simulink model "SalirClaseConObstaculos"  (R2022b)
settings: Solver=FixedStepAuto  StartTime=0.0  StopTime=inf  RelTol=1e-3  EnableMultiTasking=on
model workspace (MAT data in the model file):
  d = Simulink.Parameter
  d.Value = 0.22
  d.DataType = 'double'
  d.Complexity = 'real'
  d.Dimensions = [1 1]
libraries: robotalgslib x1
settings Model: ExtModeTrigDuration=2  Creator=Usuario_UMA  LastModifiedBy=dar.io
settings OptimizationCC: EnhancedBackFolding=on  PassReuseOutputArgsAs=Individual arguments  ZeroExternalMemoryAtStartup=off  ZeroInternalMemoryAtStartup=off  MaxStackSize=64  OptimizeBlockOrder=speed  DifferentSizesBufferReuse=on  OptimizationCustomize=off  EfficientTunableParamExpr=on
settings DebuggingCC: ParameterTunabilityLossMsg=error
settings HardwareCC: ProdBitPerInt=16  ProdBitPerPointer=16  ProdBitPerSizeT=16  ProdBitPerPtrDiffT=16  ProdLargestAtomicFloat=None  ProdWordSize=8  ProdHWDeviceType=Atmel->AVR  UseEmbeddedCoderFeatures=off  UseSimulinkCoderFeatures=off
settings SFSimCC: MATLABDynamicMemAlloc=off
settings RTWCC: Description=Embedded Coder  SystemTargetFile=ert.tlc  HardwareBoard=Arduino Mega 2560  TLCOptions=-aInlineSetEventsForThisBaseRateFcn=TLC_FALSE -aSuppressMultiTaskScheduler=TLC_FALSE -aRateBasedStepFcn=1  TemplateMakefile=ert_default_tmf  Toolchain=Arduino AVR  BuildConfiguration=Faster Runs
settings CodeAppCC: ForceParamTrailComments=on  IgnoreCustomStorageClasses=off  OperatorAnnotations=on  SimulinkDataObjDesc=on  SFDataObjDesc=on  MangleLength=10  InsertBlockDesc=on
settings ERTTargetCC: SupportContinuousTime=on  SupportNonInlinedSFcns=on  SupportVariableSizeSignals=on  ExtModeTransport=3  ExtModeStaticAlloc=on  ExtModeAutomaticAllocSize=off  ExtModeStaticAllocSize=2048  ExtModeMexFile=ext_xcp  ExtModeIntrfLevel=Level2 - Open

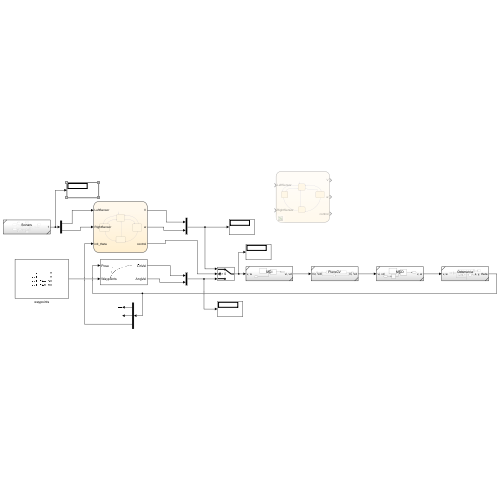
[thumbnail: Simulink's stored preview of the top-level diagram]
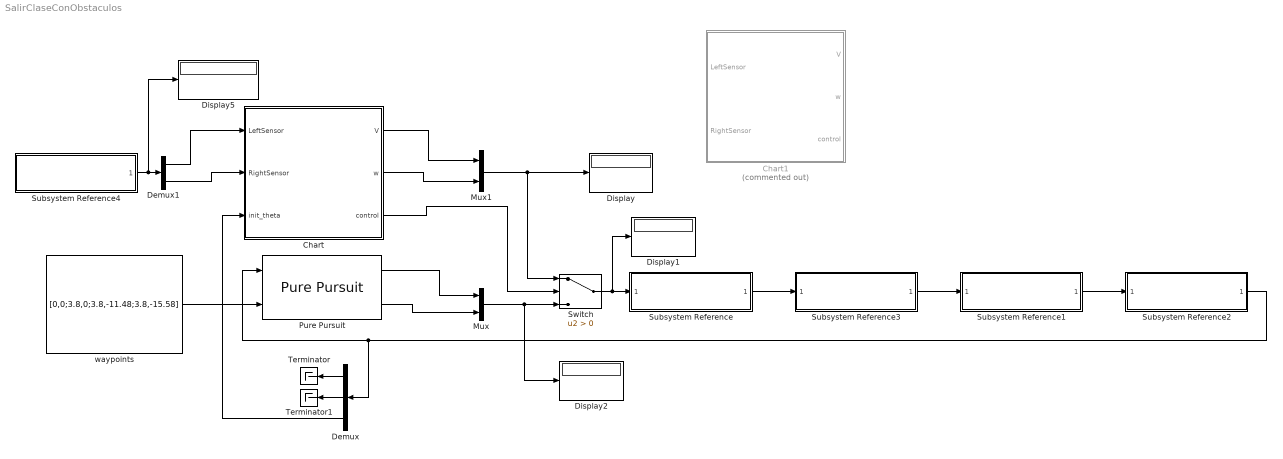
== system SalirClaseConObstaculos ==
  Chart : Stateflow chart  TreatAsAtomicUnit=on
  Chart1 : Stateflow chart  Commented=on  TreatAsAtomicUnit=on
  Demux : Demux  Outputs=3
  Demux1 : Demux  Outputs=2
  Display{,1..2,5} (4 alike) : Display
  Mux : Mux  Inputs=2
  Mux1 : Mux  Inputs=2
  Pure Pursuit : robotalgslib/Pure Pursuit  DesiredLinearVelocity=0.2  MaxAngularVelocity=1.0  LookaheadDistance=0.20  TargetDirPort=off  SimulateUsing=Code generation
      settings: LibrarySourceBlock=navlib/Control Algorithms/Pure Pursuit
  Subsystem Reference : Subsystem  ReferencedSubsystem=MCI
  Subsystem Reference1 : Subsystem  ReferencedSubsystem=MCD
  Subsystem Reference2 : Subsystem  ReferencedSubsystem=Odometria
  Subsystem Reference3 : Subsystem  ReferencedSubsystem=PieroCV
  Subsystem Reference4 : Subsystem  ReferencedSubsystem=Sonars
  Switch : Switch  Criteria=u2 > Threshold  OutDataTypeStr=double  SaturateOnIntegerOverflow=off  InputSameDT=off
  Terminator : Terminator
  Terminator1 : Terminator
  waypoints : Constant  Value=[0,0;3.8,0;3.8,-11.48;3.8,-15.58]
  wires:
  Pure Pursuit/2 -> Mux/2
  Subsystem Reference3/1 -> Subsystem Reference1/1
  Demux/2 -> Terminator1/1
  Subsystem Reference2/1 -> Demux/1, Pure Pursuit/1
  Demux/1 -> Terminator/1
  Subsystem Reference1/1 -> Subsystem Reference2/1
  Subsystem Reference/1 -> Subsystem Reference3/1
  Pure Pursuit/1 -> Mux/1
  waypoints/1 -> Pure Pursuit/2
  Chart/1(V) -> Mux1/1
  Chart/2(w) -> Mux1/2
  Mux1/1 -> Switch/1, Display/1
  Mux/1 -> Display2/1, Switch/3
  Chart/3(control) -> Switch/2
  Subsystem Reference4/1 -> Display5/1, Demux1/1
  Demux1/1 -> Chart/1(LeftSensor)
  Demux1/2 -> Chart/2(RightSensor)
  Switch/1 -> Display1/1, Subsystem Reference/1
  Demux/3 -> Chart/3(init_theta)

== stateflow chart SalirClaseConObstaculos/Chart1 ==
  state SinObstaculos
    en:
    control = 0;
    V = 0.205;
    w = 0;
  state ObstaculoIzq
    en:
    control = 1;
    V = 0.1;
    w = -0.5;
  state ObstaculoDcha
    en:
    control = 1;
    V = 0.1;
    w = 0.5;
  state ObstaculoFrente
    en:
    control = 1;
    V = 0;
    w = 0;
  (default) -> SinObstaculos
  ObstaculoDcha -> SinObstaculos [order 2] : after(3,sec)
  SinObstaculos -> ObstaculoIzq [order 1] : [LeftSensor<0.3]
  ObstaculoIzq -> SinObstaculos [order 1] : after(3,sec)
  SinObstaculos -> ObstaculoDcha [order 2] : [RightSensor<0.3]
  ObstaculoFrente -> SinObstaculos : after(3,sec)
  ObstaculoIzq -> ObstaculoFrente [order 2] : [RightSensor<0.3]
  ObstaculoDcha -> ObstaculoFrente [order 1] : [LeftSensor<0.3]
  data: LeftSensor input size=1; RightSensor input size=1; V output; w output; control output uint8 size=1

== stateflow chart SalirClaseConObstaculos/Chart ==
  state SinObstaculos
    en:
    control = 0;
    V = 0.205;
    w = 0;
  state ObstaculoDcha
    en:
    control = 1;
    V = 0.2;
    w = init_theta + pi/4;
  state ObstaculoIzq
    en:
    control = 1;
    V = 0.2;
    w = init_theta - pi/4;
  state ObstaculoFrente
    en:
    control = 1;
    V = 0;
    w = init_theta - pi/2;
  (default) -> SinObstaculos
  ObstaculoDcha -> SinObstaculos [order 2] : after(1,sec)
  SinObstaculos -> ObstaculoIzq [order 1] : [LeftSensor<0.25]
  SinObstaculos -> ObstaculoDcha [order 2] : [RightSensor<0.25]
  ObstaculoIzq -> SinObstaculos [order 1] : after(1,sec)
  ObstaculoFrente -> SinObstaculos : after(1,sec)
  ObstaculoDcha -> ObstaculoFrente [order 1] : [LeftSensor<0.25]
  ObstaculoIzq -> ObstaculoFrente [order 2] : [RightSensor<0.25]
  data: LeftSensor input size=1; RightSensor input size=1; V output; w output; control output uint8 size=1; init_theta input
